simulink model "slx1_step11_obs-1"  (R2017b)
settings: Solver=VariableStepAuto  StartTime=0.0  StopTime=10.0  RelTol=1e-3
values from neighbouring files (symbols this model uses):
  A = sys.A    [fn6_state_estimator-1.m]    (also in fn7_feedback-1.m; fn8_obsv_feedback-1.m; main_function-1.m = [a11 a12 a13 a14)
  B = sys.B    [fn6_state_estimator-1.m]    (also in fn7_feedback-1.m; fn8_obsv_feedback-1.m; main_function-1.m = [0)
  C = sys.C    [fn6_state_estimator-1.m]    (also in fn7_feedback-1.m; fn8_obsv_feedback-1.m; main_function-1.m = eye(size(A)))
  D = sys.D    [fn6_state_estimator-1.m]    (also in fn7_feedback-1.m; fn8_obsv_feedback-1.m; main_function-1.m = zeros(size(B)))
  L = transpose(L)    [fn6_state_estimator-1.m]    (also in main_function-1.m = fn6_state_estimator(sys_ss,P1,xini,xinihat))
  xini = [0;0;0;0]    [main_function-1.m]
settings Model: Creator=rakeshcm  LastModifiedBy=anusha7

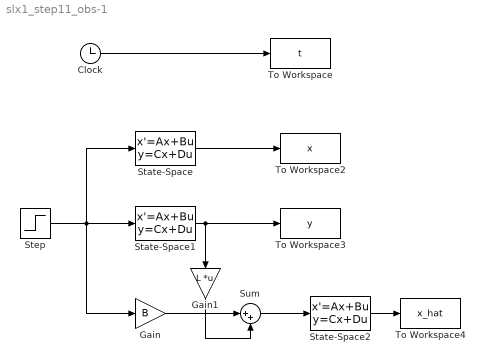
== system slx1_step11_obs-1 ==
  Clock : Clock
  Gain : Gain  Gain=B
  Gain1 : Gain  Gain=L  Multiplication=Matrix(K*u)
  State-Space : StateSpace  A=A  B=B  C=eye(size(A))  D=zeros(size(C,1),size(B,2))  InitialCondition=xini
  State-Space1 : StateSpace  A=A  B=B  C=C  D=D  InitialCondition=xini
  State-Space2 : StateSpace  A=A-L*C  B=eye(4)  C=eye(4)  D=zeros(4,4)  InitialCondition=xini
  Step : Step  Time=0  SampleTime=0
  Sum : Sum  Inputs=|++
  To Workspace : ToWorkspace  VariableName=t  SampleTime=-1
  To Workspace2 : ToWorkspace  VariableName=x  SampleTime=-1
  To Workspace3 : ToWorkspace  VariableName=y  SampleTime=-1
  To Workspace4 : ToWorkspace  VariableName=x_hat  SampleTime=-1
  wires:
  Clock/1 -> To Workspace/1
  Step/1 -> Gain/1, State-Space/1, State-Space1/1
  State-Space/1 -> To Workspace2/1
  State-Space1/1 -> To Workspace3/1, Gain1/1
  Gain/1 -> Sum/1
  Sum/1 -> State-Space2/1
  State-Space2/1 -> To Workspace4/1
  Gain1/1 -> Sum/2
